simulink model "ramadan_2022"  (R2021a)
settings: Solver=ode15s  StartTime=0.0  StopTime=10  MaxStep=1e-2  MinStep=1e-20  RelTol=1e-3
StartFcn:
  | tic
StopFcn:
  | toc
  | 
  | 
  | %if GimbalLockFlag
  |  % fprintf(2, 'Almost reached Gimbal Lock of IMU. Simulation stopped.\n')
  | %end
  | 
  | %fprintf('Elapsed time: %4.2f sec (%4.2f%% realtime)\n', a, tout(end)/a*100)
values from neighbouring files (symbols this model uses):
  Balance = pMod(26:29)    [AssignSimulinkParams.m]    (also in assign_parameters.m = param(26:29))
  BalanceTrunkLat = pMod(22:25)    [AssignSimulinkParams.m]    (also in assign_parameters.m = param(22:25))
  BasisStim = pMod(1:11)    [AssignSimulinkParams.m]    (also in assign_parameters.m = param(1:11))
  CompliantLeg = pMod(12:14)    [AssignSimulinkParams.m]    (also in assign_parameters.m = param(12:14))
  CompliantLegLat = pMod(15)    [AssignSimulinkParams.m]    (also in assign_parameters.m = param(15))
  lp1 = 0.45    [nms3D_prep.m]
  lp2 = 0.55    [nms3D_prep.m]
  N = size(x,1)    [cmaes_hg.m]
  PreventKneeOverextension = pMod(16:21)    [AssignSimulinkParams.m]    (also in assign_parameters.m = param(16:21))
  propulsion = pMod(35)    [AssignSimulinkParams.m]    (also in assign_parameters.m = param(35))
  s = x(1:N-1,:).^2 + x(2:N,:).^2    [cmaes_hg.m]
  Target02 = pMod(30)    [AssignSimulinkParams.m]    (also in assign_parameters.m = param(30))
  Target13 = pMod(31:33)    [AssignSimulinkParams.m]    (also in assign_parameters.m = param(31:33))
  theta0 = pMod(34)    [AssignSimulinkParams.m]    (also in assign_parameters.m = param(34))
  WramameiSL_1000 = readmatrix('WSL_1000_Norm_Sigmoid_MSE_cont.csv')    [nms3D_prep.m]
  ZramameiSL_1000 = readmatrix('ZSL_1000_Norm_Sigmoid_MSE_cont.csv')    [nms3D_prep.m]
undefined symbols (not defined in the file or in its folder): ICs, mParams, X, Y, Z
libraries: nesl_utility x110, sm_lib x88, simulink x79, eeGeneralControl x28, robotmaniplib x10, dspinverses x10, robotcorelib x5, dspmathops x3, pid_lib x2, vrlib x1
(part 3 of 9)

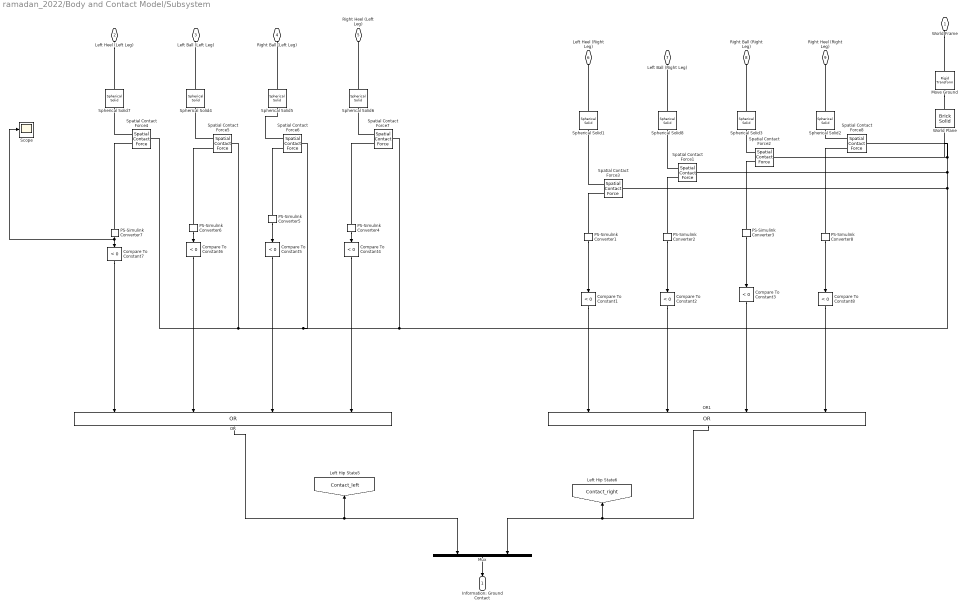
== system ramadan_2022/Body and Contact Model/Subsystem ==
  Compare To Constant{1..8} (8 alike) : simulink/Logic and Bit Operations/Compare To Constant  relop=<  const=0  OutDataTypeStr=boolean
  Move Ground : sm_lib/Frames and Transforms/Rigid Transform  TranslationMethod=StandardAxis  TranslationStandardOffset=-0.05  TranslationLengthUnit=m  TranslationStandardAxis=+Y  TranslationCartesianOffset=0  TranslationROffset=0  TranslationROffsetUnits=m  TranslationZOffset=0  TranslationZOffsetUnits=m  TranslationThetaOffset=0  TranslationThetaOffsetUnits=deg  RotationMethod=None  RotationAngleUnits=deg  RotationStandardAxis=+X  RotationAngle=-90  RotationArbitraryAxis=[0 0 1]  FollAlignAxisA=+X  BaseAlignAxisA=+Y  FollAlignAxisB=+Y  BaseAlignAxisB=+Z  RotationSequenceAxes=BaseAxes  RotationSequence=ZXZ  RotationSequenceAngles=[180 0 0]  RotationSequenceAnglesUnits=deg  RotationMatrix=[1 0 0; 0 1 0; 0 0 1]
  Mux : Mux  Inputs=2
  OR : Logic  Operator=OR  Inputs=4  AllPortsSameDT=off  OutDataTypeStr=boolean
  OR1 : Logic  Operator=OR  Inputs=4  AllPortsSameDT=off  OutDataTypeStr=boolean
  PS-Simulink Converter{1..8} (8 alike) : nesl_utility/PS-Simulink Converter  PhysicalDomain=network_engine_domain  SubClassName=ps_output  LeftPortType=input  RightPortType=output  PseudoPeriodic=off  Frequencies=[]  Unit=m  AffineConversion=off
      settings: SourceProductBaseCode=PW,SS
  Scope : Scope
  Spatial Contact Force{1..8} (8 alike) : sm_lib/Forces and Torques/Spatial Contact Force  CoefficientOfDynamicFriction=mParams.Contacts.mu_k  CoefficientOfStaticFriction=mParams.Contacts.mu_s  SenseContactBaseRotation=off  SenseContactBaseTranslation=off  NormalDamping=mParams.Contacts.damping  NormalDampingUnits=N/(m/s)  SenseContactFollowerRotation=off  SenseContactFollowerTranslation=off  SenseContactSignal=off  NormalStiffness=mParams.Contacts.stiffness  NormalStiffnessUnits=N/m  FrictionalCriticalVelocity=mParams.Contacts.vLimit  FrictionalCriticalVelocityUnits=m/s  ZeroCrossDetectContactStartAndEnd=off  FrictionType=SmoothStickSlip  SenseFrictionalForceMagnitude=off  SenseNormalForceMagnitude=off  NormalForceType=SmoothSpringDamper  SenseNormalVelocity=off  SenseSeparationDistance=on  SenseTangentialVelocity=off  SenseTangentialVelocityMagnitude=off  NormalTransitionRegionWidth=mParams.Contacts.depths  NormalTransitionRegionWidthUnits=m
  Spherical Solid{1..8} (8 alike) : sm_lib/Body Elements/Spherical Solid  GraphicAmbientColor=[0.15 0.15 0.15 1.0]  BasedOnType=Mass  CenterOfMass=[0 0 0]  CenterOfMassUnits=m  GraphicDiffuseColor=[0.5 0.5 0.5]  Density=1000  DensityUnits=kg/m^3  DoExposeReferenceFrame=on  GraphicEmissiveColor=[0.0 0.0 0.0 1.0]  ExportEntireGeometry=on  SerializedExposedGeometries=<ExposedGeometries><ExposedGeometry><RawGeometryId>entire</RawGeometryId><ExposedGeometryId>G</ExposedGeometryId></ExposedGeometry></ExposedGeometries>  SerializedFrames=<Frames/>  MarkerShape=Sphere  MarkerSize=10  GraphicType=FromGeometry  InertiaType=CalculateFromGeometry  Mass=1  MassUnits=g  MomentsOfInertia=[1 1 1]  MomentsOfInertiaUnits=kg*m^2  GraphicOpacity=1.0  ProductsOfInertia=[0 0 0]  ProductsOfInertiaUnits=kg*m^2  GraphicShininess=75  GraphicSpecularColor=[0.5 0.5 0.5 1.0]  SphereRadius=mParams.Contacts.size  SphereRadiusUnits=m  GraphicVisPropType=SimpleVisualProperties
  World Plane : sm_lib/Body Elements/Brick Solid  GraphicAmbientColor=[0.15 0.15 0.15 1.0]  BasedOnType=Density  BrickDimensions=[400 0.1 100]  BrickDimensionUnits=m  CenterOfMass=[0 0 0]  CenterOfMassUnits=m  GraphicDiffuseColor=[1.0 1.0 0.8]  Density=1000  DensityUnits=kg/(m^3)  DoExposeReferenceFrame=on  GraphicEmissiveColor=[0.0 0.0 0.0 1.0]  ExportEntireGeometry=on  SerializedFrames=<Frames/>  MarkerShape=Sphere  MarkerSize=10  GraphicType=FromGeometry  InertiaType=CalculateFromGeometry  Mass=1  MassUnits=kg  MomentsOfInertia=[1 1 1]  MomentsOfInertiaUnits=kg*m^2  GraphicOpacity=0.5  ProductsOfInertia=[0 0 0]  ProductsOfInertiaUnits=kg*m^2  GraphicShininess=75  GraphicSpecularColor=[0.5 0.5 0.5 1.0]  GraphicVisPropType=SimpleVisualProperties
  World Frame : PMIOPort  Side=Left
  Left Heel (Left Leg) : PMIOPort  Port=2  Side=Right
  Left Ball (Left Leg) : PMIOPort  Port=3  Side=Right
  Right Ball (Left Leg) : PMIOPort  Port=4  Side=Right
  Right Heel (Left Leg) : PMIOPort  Port=5  Side=Right
  Left Heel (Right Leg) : PMIOPort  Port=6  Side=Right
  Left Ball (Right Leg) : PMIOPort  Port=7  Side=Right
  Right Ball (Right Leg) : PMIOPort  Port=8  Side=Right
  Right Heel (Right Leg) : PMIOPort  Port=9  Side=Right
  Information: Ground Contact : Outport
  tag scope: Contact_left=global, Contact_right=global
  wires:
  Compare To Constant1/1 -> OR1/1
  PS-Simulink Converter4/1 -> Compare To Constant4/1
  PS-Simulink Converter5/1 -> Compare To Constant5/1
  Compare To Constant4/1 -> OR/4
  PS-Simulink Converter3/1 -> Compare To Constant3/1
  Compare To Constant6/1 -> OR/2
  PS-Simulink Converter1/1 -> Compare To Constant1/1
  PS-Simulink Converter8/1 -> Compare To Constant8/1
  Compare To Constant3/1 -> OR1/3
  Compare To Constant8/1 -> OR1/4
  PS-Simulink Converter6/1 -> Compare To Constant6/1
  PS-Simulink Converter7/1 -> Scope/1, Compare To Constant7/1
  Compare To Constant2/1 -> OR1/2
  Compare To Constant5/1 -> OR/3
  Compare To Constant7/1 -> OR/1
  PS-Simulink Converter2/1 -> Compare To Constant2/1
  OR1/1 -> [Contact_right], Mux/2
  Mux/1 -> Information: Ground Contact/1
  OR/1 -> Mux/1, [Contact_left]
  connections:
  Spatial Contact Force7/RConn1 -- Spherical Solid6/LConn1
  Spatial Contact Force5/RConn2 -- PS-Simulink Converter6/LConn1
  Spatial Contact Force1/RConn2 -- PS-Simulink Converter2/LConn1
  Spatial Contact Force7/RConn2 -- PS-Simulink Converter4/LConn1
  Spherical Solid5/RConn1 -- Right Ball (Left Leg)/RConn1
  Spatial Contact Force1/RConn1 -- Spherical Solid8/LConn1
  Spatial Contact Force2/RConn2 -- PS-Simulink Converter3/LConn1
  Spatial Contact Force8/RConn2 -- PS-Simulink Converter8/LConn1
  Spatial Contact Force6/RConn1 -- Spherical Solid5/LConn1
  Spatial Contact Force3/RConn2 -- PS-Simulink Converter1/LConn1
  Spatial Contact Force8/LConn1 -- World Plane/LConn1 -- Spatial Contact Force2/LConn1 -- Spatial Contact Force1/LConn1 -- Spatial Contact Force3/LConn1 -- Spatial Contact Force7/LConn1 -- Spatial Contact Force6/LConn1 -- Spatial Contact Force4/LConn1 -- Spatial Contact Force5/LConn1
  Spatial Contact Force5/RConn1 -- Spherical Solid4/LConn1
  Spatial Contact Force6/RConn2 -- PS-Simulink Converter5/LConn1
  Spatial Contact Force2/RConn1 -- Spherical Solid3/LConn1
  Move Ground/RConn1 -- World Plane/RConn1
  World Frame/RConn1 -- Move Ground/LConn1
  Spatial Contact Force3/RConn1 -- Spherical Solid1/LConn1
  Spherical Solid6/RConn1 -- Right Heel (Left Leg)/RConn1
  Spatial Contact Force4/RConn2 -- PS-Simulink Converter7/LConn1
  Spatial Contact Force4/RConn1 -- Spherical Solid7/LConn1
  Spherical Solid4/RConn1 -- Left Ball (Left Leg)/RConn1
  Spatial Contact Force8/RConn1 -- Spherical Solid2/LConn1
  Left Heel (Left Leg)/RConn1 -- Spherical Solid7/RConn1
  Spherical Solid2/RConn1 -- Right Heel (Right Leg)/RConn1
  Spherical Solid1/RConn1 -- Left Heel (Right Leg)/RConn1
  Spherical Solid3/RConn1 -- Right Ball (Right Leg)/RConn1
  Spherical Solid8/RConn1 -- Left Ball (Right Leg)/RConn1

== system ramadan_2022/Body and Contact Model/Trunk (floating base) ==
  Solid : sm_lib/Body Elements/Brick Solid  GraphicAmbientColor=[0.15 0.15 0.15 1.0]  BasedOnType=Density  BrickDimensions=[mParams.bodies.trunk.d mParams.bodies.trunk.l mParams.bodies.trunk.b]  BrickDimensionUnits=m  CenterOfMass=mParams.bodies.trunk.CG  CenterOfMassUnits=m  GraphicDiffuseColor=[0.5 1 0.5]  Density=2.7  DensityUnits=g/cm^3  DoExposeReferenceFrame=on  GraphicEmissiveColor=[0 0 0 1.0]  ExportEntireGeometry=off  SerializedFrames=<Frames><Frame><Id>Frame1</Id><Value><Name>CG</Name><Origin><Source>CenterOfMassFrame</Source><FeatureName></FeatureName></Origin><PrimaryAxis><DefinedDirection>+Z</DefinedDirection><Source>ReferenceFrame</Source><SourceDirection>+Z</SourceDirection><FeatureName></FeatureName></PrimaryAxis><SecondaryAxis><DefinedDirection>+X</DefinedDirection><Source>ReferenceFrame</Source><SourceDirection>+X</SourceDirection><FeatureName></FeatureName></SecondaryAxis></Value></Frame></Frames>  MarkerShape=Cube  MarkerSize=100  GraphicType=FromGeometry  InertiaType=Custom  Mass=mParams.bodies.trunk.m  MassUnits=kg  MomentsOfInertia=mParams.bodies.trunk.In  MomentsOfInertiaUnits=kg*m^2  GraphicOpacity=0.5  ProductsOfInertia=[0 0 0]  ProductsOfInertiaUnits=kg*m^2  GraphicShininess=75  GraphicSpecularColor=[0.5 0.5 0.5 1.0]  GraphicVisPropType=SimpleVisualProperties
  Transform CG to LH : sm_lib/Frames and Transforms/Rigid Transform  TranslationMethod=Cartesian  TranslationStandardOffset=0  TranslationLengthUnit=m  TranslationStandardAxis=+Y  TranslationCartesianOffset=mParams.bodies.trunk.CG_LH  TranslationROffset=0  TranslationROffsetUnits=m  TranslationZOffset=0  TranslationZOffsetUnits=m  TranslationThetaOffset=0  TranslationThetaOffsetUnits=deg  RotationMethod=None  RotationAngleUnits=deg  RotationStandardAxis=+X  RotationAngle=90  RotationArbitraryAxis=[0 0 1]  FollAlignAxisA=+X  BaseAlignAxisA=+Y  FollAlignAxisB=+Y  BaseAlignAxisB=+Z  RotationSequenceAxes=FollowerAxes  RotationSequence=XYX  RotationSequenceAngles=[0 0 0]  RotationSequenceAnglesUnits=deg  RotationMatrix=[1 0 0; 0 1 0; 0 0 1]
  Transform CG to RH : sm_lib/Frames and Transforms/Rigid Transform  TranslationMethod=Cartesian  TranslationStandardOffset=-0  TranslationLengthUnit=m  TranslationStandardAxis=+Y  TranslationCartesianOffset=mParams.bodies.trunk.CG_RH  TranslationROffset=0  TranslationROffsetUnits=m  TranslationZOffset=0  TranslationZOffsetUnits=m  TranslationThetaOffset=0  TranslationThetaOffsetUnits=deg  RotationMethod=None  RotationAngleUnits=deg  RotationStandardAxis=+X  RotationAngle=90  RotationArbitraryAxis=[0 0 1]  FollAlignAxisA=+X  BaseAlignAxisA=+Y  FollAlignAxisB=+Y  BaseAlignAxisB=+Z  RotationSequenceAxes=FollowerAxes  RotationSequence=XYX  RotationSequenceAngles=[0 0 0]  RotationSequenceAnglesUnits=deg  RotationMatrix=[1 0 0; 0 1 0; 0 0 1]
  CG : PMIOPort  Side=Left
  Left Hip : PMIOPort  Port=2  Side=Right
  Right Hip : PMIOPort  Port=3  Side=Right
  connections:
  Solid/LConn1 -- Transform CG to RH/LConn1 -- Transform CG to LH/LConn1 -- CG/RConn1
  Left Hip/RConn1 -- Transform CG to LH/RConn1
  Right Hip/RConn1 -- Transform CG to RH/RConn1

== system ramadan_2022/Body and Contact Model/Vestibular System ==
  Ankle Position Right [m] : Inport
  Ankle Position Left [m] : Inport  Port=2
  "  XYZ Sensor Left Hip" : Subsystem
  "  XYZ Sensor Right Hip" : Subsystem
  Align Axis : Subsystem
  Compare To Constant : simulink/Logic and Bit Operations/Compare To Constant  relop=<=  const=1  OutDataTypeStr=boolean
  Filtered Derivative (Discrete or Continuous) : eeGeneralControl/Filtered Derivative (Discrete or Continuous)  K=1  T=0.01  B=inf  A=-inf  minRatio=10  init_option=Inherited from block input  x0=0  Ts=0
      settings: SourceProductBaseCode=PS
  Mux : Mux  Inputs=7
  R Movement direction : Subsystem
  Scope : Scope
  Scope1 : Scope
  Selector : Selector  InputPortWidth=3  IndexOptions=Index vector (dialog)  Indices=[2]  OutputSizes=1
  Stop Simulation : Stop
  Terminator : Terminator
  Terminator1 : Terminator
  To Workspace1 : ToWorkspace  VariableName=SensorBodyFrame  SampleTime=-1
      settings: Save2DSignal=2-D array (concatenate along first dimension)
  To Workspace2 : ToWorkspace  VariableName=xyzHAT  SampleTime=-1
      settings: Save2DSignal=2-D array (concatenate along first dimension)
  "Trunk Sensor " : Subsystem
  frame : PMIOPort  Side=Left
  Right Hip : PMIOPort  Port=2  Side=Left
  Left Hip : PMIOPort  Port=3  Side=Left
  tag scope: AnklePosL_rot=global, AnklePosR_rot=global, CoM_Position=global, CoM_Velocity=global, CoM_Velocity_rot=global, HeelPosL_rot=global, HeelPosR_rot=global, HipL=global, HipR=global, R_body=global, RotationTrunk=global, RotationVelocityTrunk=global, TRK_CG=global, TrunkRotVel_lat=global, TrunkRotVel_sag=global, TrunkRot_lat=global, TrunkRot_sag=global
  wires:
  Selector/1 -> Compare To Constant/1
  Compare To Constant/1 -> Stop Simulation/1
  "Trunk Sensor "/2(Velocity Trunk [m/s]) -> Align Axis/5(Velocity Trunk [m/s]), Scope/1, Filtered Derivative (Discrete or Continuous)/1, [CoM_Velocity]
  "Trunk Sensor "/4(Rotation Trunk [rad]) -> [RotationTrunk]
  Ankle Position Right [m]/1 -> Align Axis/1(Ankle Position Right [m])
  "  XYZ Sensor Right Hip"/1(Hip Position [m]) -> [HipR], R Movement direction/1(Hip Right), Align Axis/7(Hip Position Right [m])
  R Movement direction/1("R ") -> [R_body], Align Axis/3("R ")
  Ankle Position Left [m]/1 -> Align Axis/2(Ankle Position Left [m])
  "Trunk Sensor "/1(Position Trunk [m]) -> [TRK_CG], Selector/1, To Workspace2/1, Align Axis/4(Position Trunk [m]), [CoM_Position]
  "  XYZ Sensor Left Hip"/1(Hip Position [m]) -> [HipL], Align Axis/6(Hip Position Left [m]), R Movement direction/2(Hip Left)
  "Trunk Sensor "/3(Rotation Velocity Trunk [rad/s]) -> [RotationVelocityTrunk]
  Mux/1 -> To Workspace1/1
  "  XYZ Sensor Right Hip"/2(Hip Velocity [m/s]) -> Terminator/1
  "  XYZ Sensor Left Hip"/2(Hip Velocity [m/s]) -> Terminator1/1
  Align Axis/1(Ankle Position Left (body frame)) -> [AnklePosL_rot], Mux/1
  Align Axis/2(Ankle Position Right (body frame)) -> Scope1/1, [AnklePosR_rot], Mux/2
  Align Axis/3(Trunk Velocity (body frame)) -> [CoM_Velocity_rot], Mux/3
  Align Axis/4(Saggital Trunk Rotation [rad] (body frame)) -> [TrunkRot_sag], Mux/4
  Align Axis/5(Lateral Trunk Rotation [rad] (body frame)) -> [TrunkRot_lat], Mux/5
  Align Axis/6(Saggital Trunk Rotation Velocity [rad/s] (body frame)) -> [TrunkRotVel_sag], Mux/6
  Align Axis/7(Lateral Trunk Rotation Velocity [rad/s] (body frame)) -> [TrunkRotVel_lat], Mux/7
  Align Axis/8(Heel Position Left (body frame)) -> [HeelPosL_rot]
  Align Axis/9(Heel Position Right (body frame)) -> [HeelPosR_rot]
  connections:
  "Trunk Sensor "/LConn1 -- frame/RConn1
  "  XYZ Sensor Left Hip"/LConn1 -- Left Hip/RConn1
  "  XYZ Sensor Right Hip"/LConn1 -- Right Hip/RConn1

== system ramadan_2022/Body and Contact Model/World Frame ==
  Mechanism Configuration : sm_lib/Utilities/Mechanism Configuration  UniformGravity=Constant  GravityVector=[0 -9.81 0]  GravityVectorUnits=m/s^2  GravityUnits=m/s^2  LinearizationDelta=0.001  JointModeTransitionNonlinearIterations=2
  Solver Configuration : nesl_utility/Solver Configuration  PhysicalDomain=network_engine_domain  SubClassName=solver  LeftPortType=input  RightPortType=generic  Tones=[]  Harmonics=[]  SimulateNoise=off  Profile=off  UseLocalSampling=off  EnableSwitchedLinearOptims=on  FrequencyDomain=off  UseCCode=off  RelTol=0.001  AbsTol=1e-06  MinStep=1e-09  ToWorkspace=off  RevertToSquareIcSolve=off  NumHomotopyIterations=100  PhasorMode=off  PhasorModeNumHarmonics=1  DoDC=off  ResidualTolerance=1e-9  UseLocalSolver=off  LocalSolverChoice=NE_BACKWARD_EULER_ADVANCER  LocalSolverSampleTime=.001  DoFixedCost=off  MaxNonlinIter=3  MaxModeIter=2  ComputeImpulses=off  ImpulseIterations=2  LinearAlgebra=Sparse  EquationFormulation=NE_TIME_EF  DelaysMemoryBudget=1024  AutomaticFiltering=on  FilteringTimeConstant=0.001  PartitionStorageMethod=AS_NEEDED  PartitionMemoryBudget=1024  PartitionMethod=FAST
      settings: SourceProductBaseCode=PW,SS
  World Frame : sm_lib/Frames and Transforms/World Frame
  Conn1 : PMIOPort  Side=Right
  connections:
  Solver Configuration/RConn1 -- Mechanism Configuration/RConn1 -- Conn1/RConn1 -- World Frame/RConn1

== system ramadan_2022/CMA Data/SS_dist1 ==
  In1 : Inport
  Trigger : TriggerPort  VariantControl=(inherit)  ZeroCross=off
  Delay : Delay
  Delay1 : Delay  DelayLength=1
  Mux : Mux  Inputs=3
  To Current Workspace4 : ToWorkspace  VariableName=SSdist  SaveFormat=Structure With Time  SampleTime=-1
      settings: MaxDataPoints=3
  SSdist : Outport
  wires:
  In1/1 -> Delay/1, Delay1/1, Mux/3, To Current Workspace4/1
  Delay/1 -> Mux/1
  Delay1/1 -> Mux/2
  Mux/1 -> SSdist/1

== system ramadan_2022/CMA Data/SS_dist2 ==
  Steplengths : Inport
  Trigger : TriggerPort  VariantControl=(inherit)  ZeroCross=off
  Steplength at DS : Outport
  wires:
  Steplengths/1 -> Steplength at DS/1

== system ramadan_2022/CMA Data/Step Counter ==
  Step2 : Inport
  Step1 : Inport  Port=2
  Constant1 : Constant  Value=0
  Constant2 : Constant  Value=0
  Constant3 : Constant  Value=0
  Constant4 : Constant  Value=-1
  Saturation Dynamic : simulink/Discontinuities/Saturation Dynamic  OutMin=[]  OutMax=[]  OutDataTypeStr=Inherit: Same as second input  OutDataType=fixdt(1, 16)  OutScaling=2^-10  DoSatur=off
  Saturation Dynamic1 : simulink/Discontinuities/Saturation Dynamic  OutMin=[]  OutMax=[]  OutDataTypeStr=Inherit: Same as second input  OutDataType=fixdt(1, 16)  OutScaling=2^-10  DoSatur=off
  Sum : Sum  Inputs=|++
  Sum1 : Sum  Inputs=++|
  Sum2 : Sum  Inputs=|++
  count steps1 : Subsystem  TreatAsAtomicUnit=on
  count steps2 : Subsystem  TreatAsAtomicUnit=on
  nStep : Outport  VectorParamsAs1DForOutWhenUnconnected=off
  wires:
  count steps1/1(nStep) -> Saturation Dynamic1/2, Sum2/2, Sum/2
  count steps2/1(nStep) -> Saturation Dynamic/2, Sum1/1, Sum/1
  Constant3/1 -> Saturation Dynamic/3
  Saturation Dynamic/1 -> count steps2/1(nStep-1)
  Constant1/1 -> Sum1/2
  Sum1/1 -> Saturation Dynamic1/1
  Constant2/1 -> Saturation Dynamic1/3
  Saturation Dynamic1/1 -> count steps1/1(nStep-1)
  Constant4/1 -> Sum2/1
  Sum2/1 -> Saturation Dynamic/1
  Step2/1 -> count steps2/Trigger
  Sum/1 -> nStep/1
  Step1/1 -> count steps1/Trigger

== system ramadan_2022/CMA Data/Triggered Subsystem ==
  In1 : Inport
  Trigger : TriggerPort  VariantControl=Variant
  Out1 : Outport
  wires:
  In1/1 -> Out1/1

== system ramadan_2022/CMA Data/check steady state ==
  p : Inport
  nStep : Inport  Port=2
  Abs : Abs  ZeroCross=off
  Add{,1..9,15..16} (12 alike) : Sum  Inputs=-+
  Add{10..14,17} (6 alike) : Sum  Inputs=+-
  Demux2 : Demux  Outputs=7
  Demux3 : Demux  Outputs=7
  Fcn : Fcn  Expr=rem(u(1), 2)
  Gain14 : Gain  Gain=.5
  Mux1 : Mux  Inputs=6
  Rounding Function1 : Rounding
  Sum of Elements : Sum  Inputs=+
  even : Subsystem  TreatAsAtomicUnit=on
  odd : Subsystem  TreatAsAtomicUnit=on
  SS_dist : Outport  VectorParamsAs1DForOutWhenUnconnected=off
  wires:
  p/1 -> even/1(In1), odd/1(In1)
  Fcn/1 -> odd/Trigger, even/Trigger
  odd/1(Out1) -> Demux2/1
  even/1(Out1) -> Demux3/1
  Add10/1 -> Mux1/1
  Add11/1 -> Mux1/2
  Add12/1 -> Mux1/3
  Add13/1 -> Mux1/4
  Add14/1 -> Mux1/5
  Demux2/2 -> Add/2
  Demux2/3 -> Add1/2
  Demux2/4 -> Add2/2
  Demux2/5 -> Add3/2
  Demux2/6 -> Add4/2
  Demux2/1 -> Add/1, Add1/1, Add2/1, Add3/1, Add4/1, Add15/1
  Demux3/2 -> Add5/2
  Demux3/3 -> Add6/2
  Demux3/4 -> Add7/2
  Demux3/5 -> Add8/2
  Demux3/6 -> Add9/2
  Demux3/1 -> Add5/1, Add6/1, Add7/1, Add8/1, Add9/1, Add16/1
  Add/1 -> Add10/1
  Add1/1 -> Add11/1
  Add2/1 -> Add12/1
  Add3/1 -> Add13/1
  Add4/1 -> Add14/1
  Add5/1 -> Add10/2
  Add6/1 -> Add11/2
  Add7/1 -> Add12/2
  Add8/1 -> Add13/2
  Add9/1 -> Add14/2
  Mux1/1 -> Abs/1
  Abs/1 -> Sum of Elements/1
  Sum of Elements/1 -> SS_dist/1
  nStep/1 -> Gain14/1
  Gain14/1 -> Rounding Function1/1
  Rounding Function1/1 -> Fcn/1
  Demux2/7 -> Add15/2
  Demux3/7 -> Add16/2
  Add15/1 -> Add17/1
  Add16/1 -> Add17/2
  Add17/1 -> Mux1/6

== system ramadan_2022/CMA Data/mean (10s) ==
  u : Inport
  Constant : Constant  Value=1001
  Divide2 : Product  Inputs=*/
  Sum of Elements : Sum  Inputs=+  CollapseMode=Specified dimension  AccumDataTypeStr=double
  Tapped Delay : simulink/Discrete/Tapped Delay  vinit=1  samptime=0.01  NumDelays=1000  DelayOrder=Newest  includeCurrent=off
  Vector Concatenate : Concatenate
  u_average : Outport
  wires:
  Tapped Delay/1 -> Vector Concatenate/2
  Vector Concatenate/1 -> Sum of Elements/1
  Sum of Elements/1 -> Divide2/1
  Divide2/1 -> u_average/1
  u/1 -> Tapped Delay/1, Vector Concatenate/1
  Constant/1 -> Divide2/2

== system ramadan_2022/CMA Data/mean (10s)1 ==
  u : Inport
  Constant : Constant  Value=1001
  Divide2 : Product  Inputs=*/
  Sum of Elements : Sum  Inputs=+  CollapseMode=Specified dimension  AccumDataTypeStr=double
  Tapped Delay : simulink/Discrete/Tapped Delay  vinit=ICs.trunk.vx0  samptime=0.01  NumDelays=1000  DelayOrder=Newest  includeCurrent=off
  Vector Concatenate : Concatenate
  u_average : Outport
  wires:
  Tapped Delay/1 -> Vector Concatenate/2
  Vector Concatenate/1 -> Sum of Elements/1
  Sum of Elements/1 -> Divide2/1
  Divide2/1 -> u_average/1
  u/1 -> Tapped Delay/1, Vector Concatenate/1
  Constant/1 -> Divide2/2

== system ramadan_2022/CMA Data/mean (10s)2 ==
  u : Inport
  Constant : Constant  Value=1001
  Divide2 : Product  Inputs=*/
  Sum of Elements : Sum  Inputs=+  CollapseMode=Specified dimension  AccumDataTypeStr=double
  Tapped Delay : simulink/Discrete/Tapped Delay  vinit=ICs.trunk.vx0  samptime=0.001  NumDelays=1000  DelayOrder=Newest  includeCurrent=off
  Vector Concatenate : Concatenate
  u_average : Outport
  wires:
  Tapped Delay/1 -> Vector Concatenate/2
  Vector Concatenate/1 -> Sum of Elements/1
  Sum of Elements/1 -> Divide2/1
  Divide2/1 -> u_average/1
  u/1 -> Tapped Delay/1, Vector Concatenate/1
  Constant/1 -> Divide2/2

== system ramadan_2022/CMA Data/phase 1? ==
  cadence : Inport
  stability : Inport  Port=2
  AND1 : Logic  AllPortsSameDT=off  OutDataTypeStr=boolean
  AND2 : Logic  AllPortsSameDT=off  OutDataTypeStr=boolean
  Clock : Clock
  Compare To Constant : simulink/Logic and Bit Operations/Compare To Constant  relop=>=  const=30  OutDataTypeStr=boolean
  Compare To Constant1 : simulink/Logic and Bit Operations/Compare To Constant  relop=<=  const=135  OutDataTypeStr=boolean
  Compare To Constant2 : simulink/Logic and Bit Operations/Compare To Constant  relop===  const=10  OutDataTypeStr=boolean
  OR : Logic  Operator=OR  AllPortsSameDT=off  OutDataTypeStr=boolean
  Stop Simulation1 : Stop
  time : Outport
  wires:
  cadence/1 -> Compare To Constant1/1
  Compare To Constant1/1 -> AND1/1
  Compare To Constant/1 -> AND2/2
  stability/1 -> Compare To Constant/1
  Compare To Constant2/1 -> AND2/1, AND1/2
  AND2/1 -> OR/2
  AND1/1 -> OR/1
  Clock/1 -> time/1, Compare To Constant2/1
  OR/1 -> Stop Simulation1/1

== system ramadan_2022/Muscle Actuation Layer/Muscles Left ==
  STIM Left : Inport
  Demux : Demux
  Muscle Dynamics (Vectorized)1 : Subsystem
  Muscle Length Vector1 : Subsystem
  Muscle Torque Contributions1 : Subsystem
  Terminator : Terminator
  Terminator1 : Terminator
  To Workspace1 : ToWorkspace  VariableName=LForce  SampleTime=-1
      settings: Save2DSignal=2-D array (concatenate along first dimension)
  tauHipPitchL : Outport
  tauHipRollL : Outport  Port=2
  tauKneeL : Outport  Port=3
  tauHipAnkleL : Outport  Port=4
  "Leg Torque " : Outport  Port=5
  tag scope: LFmVec=global, LLceVec=global, LVceVec=global
  wires:
  Demux/2 -> Muscle Length Vector1/2(qHipRoll [rad])
  Muscle Torque Contributions1/2(tauHR [Nm]) -> tauHipRollL/1
  Demux/1 -> Muscle Length Vector1/1(qHipPitch [rad])
  Demux/4 -> Muscle Torque Contributions1/2(qAnkle [rad]), Muscle Length Vector1/4(qAnkle [rad])  "qA"
  Muscle Dynamics (Vectorized)1/3(Vce) -> [LVceVec]
  Muscle Torque Contributions1/3(tauK [Nm]) -> tauKneeL/1
  Demux/3 -> Muscle Torque Contributions1/1(qKnee [rad]), Muscle Length Vector1/3(qKnee [rad])  "qK"
  Muscle Dynamics (Vectorized)1/5(ForceLengthFactor) -> Terminator1/1
  Muscle Length Vector1/1(lmtc [m x11]) -> Muscle Dynamics (Vectorized)1/1(lmtc [m])
  Muscle Torque Contributions1/1(tauHP [Nm]) -> tauHipPitchL/1
  Muscle Torque Contributions1/4(tauA [Nm]) -> tauHipAnkleL/1
  Muscle Dynamics (Vectorized)1/4(A) -> Terminator/1
  Muscle Dynamics (Vectorized)1/2(Lce) -> [LLceVec]
  STIM Left/1 -> Muscle Dynamics (Vectorized)1/2(STIM)
  [Llegq] -> Demux/1
  Muscle Torque Contributions1/5(Leg Torque) -> "Leg Torque "/1
  Muscle Dynamics (Vectorized)1/1(Fmtc) -> To Workspace1/1, Muscle Torque Contributions1/3(FmVec [N x11]), [LFmVec]

== system ramadan_2022/Muscle Actuation Layer/Muscles Right ==
  STIM Right : Inport
  Demux : Demux
  Goto15 : Goto  Commented=on  GotoTag=activation_R  TagVisibility=global
  Muscle Dynamics (Vectorized) : Subsystem
  Muscle Length Vector : Subsystem
  Muscle Torque Contributions : Subsystem
  R Leg Muscles Vce [m/s x11]1 : Goto  Commented=on  GotoTag=RForceLength  TagVisibility=global
  To Workspace1 : ToWorkspace  VariableName=RForce  SampleTime=-1
      settings: Save2DSignal=2-D array (concatenate along first dimension)
  tauHipPitchR : Outport
  tauHipRollR : Outport  Port=2
  tauKneeR : Outport  Port=3
  tauHipAnkleR : Outport  Port=4
  Leg Torque : Outport  Port=5
  tag scope: RFmVec=global, RLceVec=global, RVceVec=global
  wires:
  Muscle Torque Contributions/4(tauA [Nm]) -> tauHipAnkleR/1
  Muscle Torque Contributions/3(tauK [Nm]) -> tauKneeR/1
  Muscle Length Vector/1(lmtc [m x11]) -> Muscle Dynamics (Vectorized)/1(lmtc [m])
  Demux/3 -> Muscle Torque Contributions/1(qKnee [rad]), Muscle Length Vector/3(qKnee [rad])  "qK"
  Demux/4 -> Muscle Torque Contributions/2(qAnkle [rad]), Muscle Length Vector/4(qAnkle [rad])  "qA"
  Muscle Dynamics (Vectorized)/2(Lce) -> [RLceVec]
  Muscle Torque Contributions/2(tauHR [Nm]) -> tauHipRollR/1
  Demux/1 -> Muscle Length Vector/1(qHipPitch [rad])  "qHP"
  Muscle Dynamics (Vectorized)/5(ForceLengthFactor) -> R Leg Muscles Vce [m/s x11]1/1
  Muscle Dynamics (Vectorized)/1(Fmtc) -> To Workspace1/1, Muscle Torque Contributions/3(FmVec [N x11]), [RFmVec]
  Muscle Dynamics (Vectorized)/4(A) -> Goto15/1
  Muscle Dynamics (Vectorized)/3(Vce) -> [RVceVec]
  Muscle Torque Contributions/1(tauHP [Nm]) -> tauHipPitchR/1
  Demux/2 -> Muscle Length Vector/2(qHipRoll [rad])  "qHR"
  STIM Right/1 -> Muscle Dynamics (Vectorized)/2(STIM)
  [Rlegq] -> Demux/1  "qHP"
  Muscle Torque Contributions/5(Leg Torque) -> Leg Torque/1

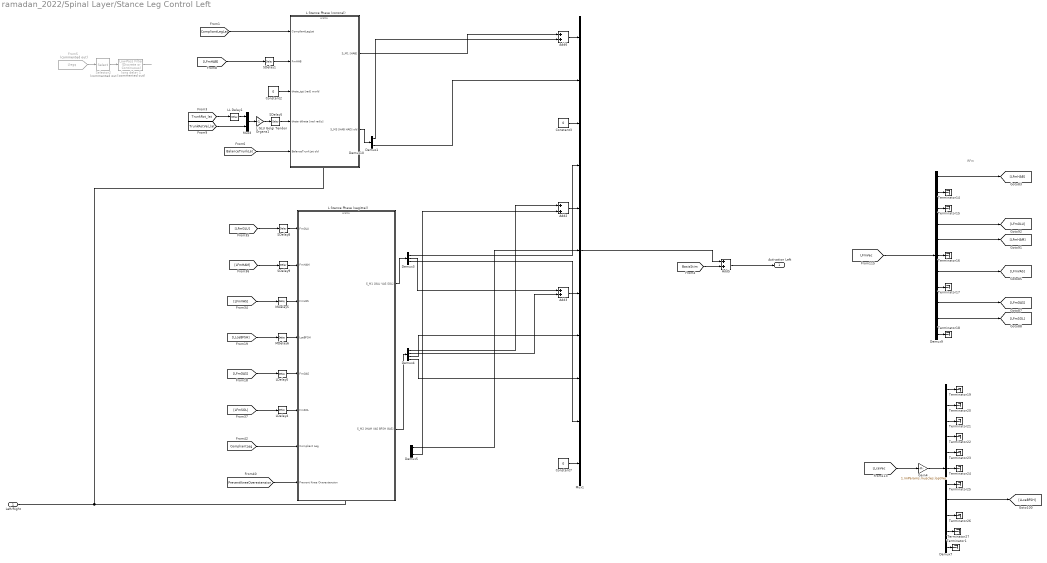
== system ramadan_2022/Spinal Layer/Stance Leg Control Left ==
  note: RFm
  Left/Right : Inport
  Add{2..3,5..6} (4 alike) : Sum
  Constant2 : Constant  Value=0
  Constant3 : Constant  Value=0
  Constant7 : Constant  Value=0
  Demux1 : Demux  Outputs=2
  Demux10 : Demux  Outputs=2
  Demux3 : Demux  Outputs=3
  Demux4 : Demux
  Demux5 : Demux  Outputs=2
  Demux7 : Demux  Outputs=11
  Demux9 : Demux  Outputs=11
  From5 : From  Commented=on  GotoTag=Llegq  TagVisibility=global
      settings: CloseFcn=tagdialog Close
  Gain4 : Gain  Gain=1./mParams.muscles.loptVec
  L GLU Golgi Tendon Organs1 : Gain  Gain=-1
  L Stance Phase (coronal) : Subsystem  TreatAsAtomicUnit=on
  L Stance Phase (sagittal) : Subsystem  TreatAsAtomicUnit=on
  LDelay4 : TransportDelay  DelayTime=mParams.control.delays.long
  LDelay5 : TransportDelay  DelayTime=mParams.control.delays.long
  LL Delay1 : TransportDelay  DelayTime=mParams.control.delays.longloop/2
  MDelay5 : TransportDelay  DelayTime=mParams.control.delays.mid
  MDelay6 : TransportDelay  DelayTime=mParams.control.delays.mid
  Mux1 : Mux  Inputs=11
  Mux3 : Mux  Inputs=2
  SDelay{1,5,8..9} (4 alike) : TransportDelay  DelayTime=mParams.control.delays.short
  Selector2 : Selector  Commented=on  InputPortWidth=4  IndexOptions=Index vector (dialog)  Indices=[2]  OutputSizes=1
  Terminator{1,14..27} (15 alike) : Terminator
  long delay 1 : eeGeneralControl/Low-Pass Filter (Discrete or Continuous)  Commented=on  K=1  T=0.005  B=inf  A=-inf  init_option=Inherited from block input  x0=0  Ts=0
  Activation Left : Outport
  wires:
  [LFmVec] -> Demux9/1
  Demux9/1 -> [LFmHAB]
  Gain4/1 -> Demux7/1
  Demux9/5 -> [LFmHAM]
  Demux7/8 -> [LLceBFSH]
  [LLceVec] -> Gain4/1
  Demux9/9 -> [LFmGAS]
  Demux9/10 -> [LFmSOL]
  Demux9/4 -> [LFmGLU]
  Demux9/7 -> [LFmVAS]
  Demux7/11 -> Terminator1/1
  Add5/1 -> Activation Left/1
  Left/Right/1 -> L Stance Phase (sagittal)/Enable, L Stance Phase (coronal)/Enable
  Demux9/2 -> Terminator14/1
  Demux9/3 -> Terminator15/1
  Demux9/6 -> Terminator16/1
  Demux9/8 -> Terminator17/1
  Demux9/11 -> Terminator18/1
  Demux7/1 -> Terminator19/1
  Demux7/2 -> Terminator20/1
  Demux7/3 -> Terminator21/1
  Demux7/4 -> Terminator22/1
  Demux7/5 -> Terminator23/1
  Demux7/6 -> Terminator24/1
  Demux7/7 -> Terminator25/1
  Demux7/9 -> Terminator26/1
  Demux7/10 -> Terminator27/1
  [BasisStim] -> Add5/2
  Mux1/1 -> Add5/1
  Constant7/1 -> Mux1/11
  Add2/1 -> Mux1/5
  Add3/1 -> Mux1/7
  [LFmGLU] -> SDelay8/1
  SDelay9/1 -> L Stance Phase (sagittal)/2(FmHAM)
  MDelay6/1 -> L Stance Phase (sagittal)/4(LceBFSH)
  [LLceBFSH] -> MDelay6/1
  [LFmSOL] -> LDelay4/1
  MDelay5/1 -> L Stance Phase (sagittal)/3(FmVAS)
  [LFmGAS] -> LDelay5/1
  LDelay5/1 -> L Stance Phase (sagittal)/5(FmGAS)
  SDelay8/1 -> L Stance Phase (sagittal)/1(FmGLU)
  [LFmHAM] -> SDelay9/1
  LDelay4/1 -> L Stance Phase (sagittal)/6(FmSOL)
  [LFmVAS] -> MDelay5/1
  [CompliantLeg] -> L Stance Phase (sagittal)/7(Compliant Leg)
  [PreventKneeOverextension] -> L Stance Phase (sagittal)/8(Prevent Knee Overextension)
  [CompliantLegLat] -> L Stance Phase (coronal)/1(CompliantLegLat)
  From5/1 -> Selector2/1
  [LFmHAB] -> SDelay1/1
  SDelay1/1 -> L Stance Phase (coronal)/2(FmHAB)
  long delay 1/1 -> ?
  Add6/1 -> Mux1/1
  Selector2/1 -> long delay 1/1
  SDelay5/1 -> L Stance Phase (coronal)/4(theta dtheta [rad rad/s])
  [TrunkRotVel_lat] -> Mux3/2
  [TrunkRot_lat] -> LL Delay1/1
  LL Delay1/1 -> Mux3/1
  [BalanceTrunkLat] -> L Stance Phase (coronal)/5(BalanceTrunkLat old)
  Mux3/1 -> L GLU Golgi Tendon Organs1/1
  L GLU Golgi Tendon Organs1/1 -> SDelay5/1
  L Stance Phase (coronal)/1(S_M1 [HAB]) -> Add6/1
  L Stance Phase (coronal)/2(S_M3 [HAB HAD] old) -> Demux1/1
  Demux1/1 -> Add6/2
  Demux1/2 -> Mux1/2
  L Stance Phase (sagittal)/1(S_M1 [GLU VAS SOL]) -> Demux3/1
  L Stance Phase (sagittal)/2(S_M2 [HAM VAS BFSH GAS]) -> Demux4/1
  ? -> Demux5/1
  Demux3/1 -> Mux1/4
  Demux4/1 -> Add2/1
  Demux5/2 -> Add2/2
  Demux5/1 -> Mux1/6
  Demux3/2 -> Add3/1
  Demux4/2 -> Add3/2
  Demux4/3 -> Mux1/8
  Demux4/4 -> Mux1/9
  Demux3/3 -> Mux1/10
  Constant2/1 -> L Stance Phase (coronal)/3(theta_tgt [rad] world)
  Constant3/1 -> Mux1/3

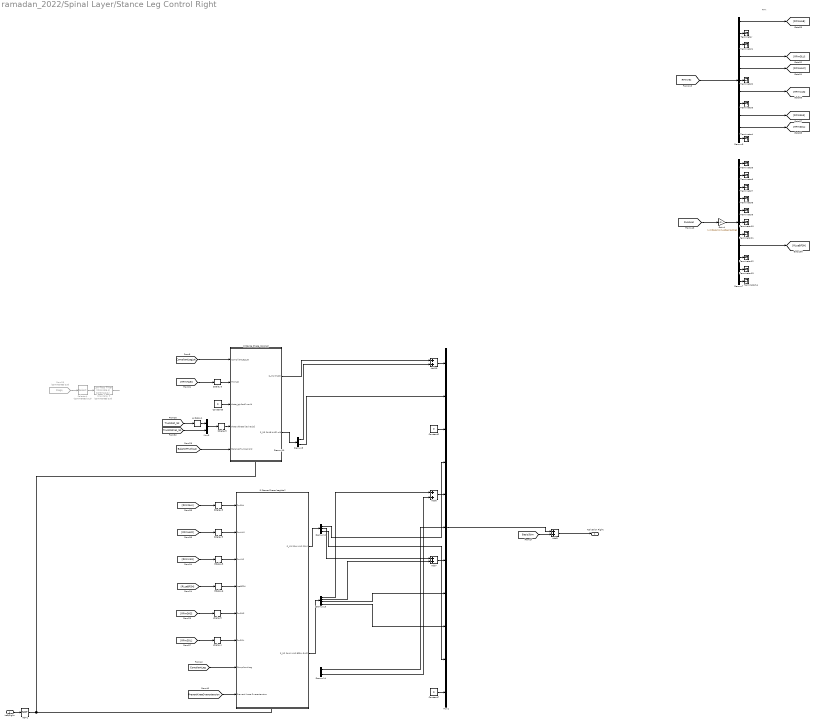
== system ramadan_2022/Spinal Layer/Stance Leg Control Right ==
  note: RFm
  Left/Right : Inport
  Add{6..7,9..10} (4 alike) : Sum
  Constant2 : Constant  Value=0
  Constant3 : Constant  Value=0
  Constant7 : Constant  Value=0
  Demux10 : Demux  Outputs=2
  Demux12 : Demux  Outputs=3
  Demux13 : Demux
  Demux14 : Demux  Outputs=2
  Demux7 : Demux  Outputs=11
  Demux8 : Demux  Outputs=2
  Demux9 : Demux  Outputs=11
  From28 : From  Commented=on  GotoTag=Rlegq  TagVisibility=global
      settings: CloseFcn=tagdialog Close
  Gain4 : Gain  Gain=1./mParams.muscles.loptVec
  LDelay4 : TransportDelay  DelayTime=mParams.control.delays.long
  LDelay5 : TransportDelay  DelayTime=mParams.control.delays.long
  LL Delay1 : TransportDelay  DelayTime=mParams.control.delays.longloop/2
  MDelay5 : TransportDelay  DelayTime=mParams.control.delays.mid
  MDelay6 : TransportDelay  DelayTime=mParams.control.delays.mid
  Mux1 : Mux  Inputs=11
  Mux3 : Mux  Inputs=2
  NOT1 : Logic  Operator=NOT  AllPortsSameDT=off  OutDataTypeStr=boolean
  R Stance Phase (coronal) : Subsystem  TreatAsAtomicUnit=on
  R Stance Phase (sagittal) : Subsystem  TreatAsAtomicUnit=on
  SDelay{3,5,8..9} (4 alike) : TransportDelay  DelayTime=mParams.control.delays.short
  Selector4 : Selector  Commented=on  InputPortWidth=4  IndexOptions=Index vector (dialog)  Indices=[2]  OutputSizes=1
  Terminator{,1..14} (15 alike) : Terminator
  long delay 3 : eeGeneralControl/Low-Pass Filter (Discrete or Continuous)  Commented=on  K=1  T=0.005  B=inf  A=-inf  init_option=Inherited from block input  x0=0  Ts=0
  Activation Right : Outport
  wires:
  [RFmVec] -> Demux9/1
  Demux9/1 -> [RFmHAB]
  Gain4/1 -> Demux7/1
  Demux9/5 -> [RFmHAM]
  Demux7/8 -> [RLceBFSH]
  Demux9/9 -> [RFmGAS]
  Demux9/10 -> [RFmSOL]
  Demux9/4 -> [RFmGLU]
  Demux9/7 -> [RFmVAS]
  Demux7/11 -> Terminator14/1
  [RLceVec] -> Gain4/1
  Demux9/2 -> Terminator/1
  Demux9/3 -> Terminator1/1
  Demux9/6 -> Terminator2/1
  Demux9/8 -> Terminator3/1
  Demux9/11 -> Terminator4/1
  Demux7/1 -> Terminator5/1
  Demux7/2 -> Terminator6/1
  Demux7/3 -> Terminator7/1
  Demux7/4 -> Terminator8/1
  Demux7/5 -> Terminator9/1
  Demux7/6 -> Terminator10/1
  Demux7/7 -> Terminator11/1
  Demux7/9 -> Terminator12/1
  Demux7/10 -> Terminator13/1
  [RFmHAB] -> SDelay3/1
  LL Delay1/1 -> Mux3/1
  [CompliantLeg] -> R Stance Phase (sagittal)/7(Compliant Leg)
  Demux13/1 -> Add6/1
  Left/Right/1 -> NOT1/1
  Demux12/2 -> Add7/1
  [RFmGLU] -> SDelay8/1
  SDelay8/1 -> R Stance Phase (sagittal)/1(FmGLU)
  [RLceBFSH] -> MDelay6/1
  Add6/1 -> Mux1/5
  Demux12/3 -> Mux1/10
  MDelay6/1 -> R Stance Phase (sagittal)/4(LceBFSH)
  Mux3/1 -> SDelay5/1
  From28/1 -> Selector4/1
  Demux13/4 -> Mux1/9
  [RFmGAS] -> LDelay5/1
  Constant7/1 -> Mux1/11
  [RFmSOL] -> LDelay4/1
  SDelay9/1 -> R Stance Phase (sagittal)/2(FmHAM)
  [TrunkRot_lat] -> LL Delay1/1
  LDelay4/1 -> R Stance Phase (sagittal)/6(FmSOL)
  [BasisStim] -> Add9/2
  Add10/1 -> Mux1/1
  Add7/1 -> Mux1/7
  Mux1/1 -> Add9/1
  Constant2/1 -> Mux1/3
  Add9/1 -> Activation Right/1
  R Stance Phase (coronal)/1(S_M1 [HAB]) -> Add10/1
  ? -> Demux14/1
  [RFmVAS] -> MDelay5/1
  Demux13/2 -> Add7/2
  Demux13/3 -> Mux1/8
  Selector4/1 -> long delay 3/1
  Demux14/2 -> Add6/2
  R Stance Phase (coronal)/2(S_M3 [HAB HAD] old) -> Demux8/1
  Demux14/1 -> Mux1/6
  Demux8/2 -> Mux1/2
  [RFmHAM] -> SDelay9/1
  Demux12/1 -> Mux1/4
  long delay 3/1 -> ?
  SDelay5/1 -> R Stance Phase (coronal)/4(theta dtheta [rad rad/s])
  R Stance Phase (sagittal)/2(S_M2 [HAM VAS BFSH GAS]) -> Demux13/1
  R Stance Phase (sagittal)/1(S_M1 [GLU VAS SOL]) -> Demux12/1
  Demux8/1 -> Add10/2
  LDelay5/1 -> R Stance Phase (sagittal)/5(FmGAS)
  [PreventKneeOverextension] -> R Stance Phase (sagittal)/8(Prevent Knee Overextension)
  MDelay5/1 -> R Stance Phase (sagittal)/3(FmVAS)
  [TrunkRotVel_lat] -> Mux3/2
  [BalanceTrunkLat] -> R Stance Phase (coronal)/5(BalanceTrunkLat old)
  [CompliantLegLat] -> R Stance Phase (coronal)/1(CompliantLegLat)
  SDelay3/1 -> R Stance Phase (coronal)/2(FmHAB)
  NOT1/1 -> R Stance Phase (sagittal)/Enable, R Stance Phase (coronal)/Enable
  Constant3/1 -> R Stance Phase (coronal)/3(theta_tgt [rad] world)

== system ramadan_2022/Spinal Layer/Stretch Reflex for Swing Leg Control ==
  Descending Commands Left : Inport
  Descending Commands Right : Inport  Port=2
  Filtered Derivative (Discrete or Continuous)1 : eeGeneralControl/Filtered Derivative (Discrete or Continuous)  K=1  T=0.0025  B=inf  A=-inf  minRatio=10  init_option=Inherited from block input  x0=0  Ts=0
      settings: SourceProductBaseCode=PS
  Filtered Derivative (Discrete or Continuous)2 : eeGeneralControl/Filtered Derivative (Discrete or Continuous)  K=1  T=0.0025  B=inf  A=-inf  minRatio=10  init_option=Inherited from block input  x0=0  Ts=0
      settings: SourceProductBaseCode=PS
  Saturation1 : Saturate  UpperLimit=1  LowerLimit=0  ZeroCross=off
  Saturation4 : Saturate  UpperLimit=1  LowerLimit=0  ZeroCross=off
  Stretch Reflex Left : Subsystem
  Stretch Reflex Right : Subsystem
  Time Delay{,1..4} (5 alike) : eeGeneralControl/Low-Pass Filter (Discrete or Continuous)  K=1  T=0.0025  B=inf  A=-inf  init_option=Inherited from block input  x0=0  Ts=0
  Time Delay5 : eeGeneralControl/Low-Pass Filter (Discrete or Continuous)  K=1  T=0.0025  B=inf  A=-inf  init_option=Inherited from block input  x0=0  Ts=-1
  Activation Left : Outport
  Activation Right : Outport  Port=2
  wires:
  Descending Commands Left/1 -> Time Delay/1, Filtered Derivative (Discrete or Continuous)2/1
  Filtered Derivative (Discrete or Continuous)1/1 -> Stretch Reflex Right/4(lambda_dot)
  Descending Commands Right/1 -> Time Delay3/1, Filtered Derivative (Discrete or Continuous)1/1
  Stretch Reflex Right/1(STIM) -> Saturation4/1
  Stretch Reflex Left/1(STIM) -> Saturation1/1
  Filtered Derivative (Discrete or Continuous)2/1 -> Stretch Reflex Left/4(lambda_dot)
  [LLceVec] -> Time Delay1/1
  [LVceVec] -> Time Delay2/1
  [RVceVec] -> Time Delay5/1
  [RLceVec] -> Time Delay4/1
  Time Delay2/1 -> Stretch Reflex Left/3(v_ce)
  Time Delay1/1 -> Stretch Reflex Left/2(l_ce)
  Time Delay/1 -> Stretch Reflex Left/1(lambda)
  Time Delay4/1 -> Stretch Reflex Right/2(l_ce)
  Time Delay5/1 -> Stretch Reflex Right/3(v_ce)
  Time Delay3/1 -> Stretch Reflex Right/1(lambda)
  Saturation1/1 -> Activation Left/1
  Saturation4/1 -> Activation Right/1

== system ramadan_2022/Supraspinal Level/Finite State Machine ==
  note: Finite State Machine (FSM): The FSM comprises 4 states (Early Right Swing (0), Late Right Swing (1), Early Left Swing (2) and Late Left Swing (3)). The FSM transitions from state 0 to state 1 and from state 2 to state 3 when the time dt in state 0/2 is passed. It transitions from state 2 to state 3 and from state 3 to state 1 when right/left contact is measured.
  Information: Ground Contact : Inport
  Chart : Stateflow chart  TreatAsAtomicUnit=on
      settings: PortSchema="{\"entries\":[{\"content\":{\"sides\":[{\"content\":{\"connectorIds\":[\"In3\",\"In4\",\"In5\"]},\"type\":\"ConnectorPlacement.EquallySpacedRectSide\",\"uuid\":\"32e0668c-48c8-429f-a891-bfe2264b7e83\"},{\"content\":{\"connectorIds\":[\"Out1\",\"Out2\",\"Out3\",\"Out4\",\"Out5\",\"Out6\"],\"side\":\"RIGHT\"},\"type\":\"ConnectorPlacement.EquallySpacedRectSide\",\"uuid\":\"eb9fc1c2-0f15-47d7-b4d3-2749cce0de04\"},{\"content\":{\"connectorIds\":[\"In1\",\"In2\"],\"side\":\"TOP\"},\"type\":\"ConnectorPlacement.EquallySpacedRectSide\",\"uuid\":\"f1bd4247-3561-4736-9dd1-6be63b5db75c\"}]},\"type\":\"ConnectorPlacement.EquallySpacedConnector\",\"uuid\":\"7da9c37e-47e6-4ed1-b08d-da72e495dbd7\"}],\"packageUris\":[\"http://schema.mathworks.com/mf0/Connector/R2020b\"],\"version\":\"1.0\"}"
  Constant : Constant  Value=lp1
  Constant1 : Constant  Value=lp2
  Demux : Demux  Outputs=2
  Early Right Swing : Outport
  Late Right Swing : Outport  Port=2
  Early Left Swing : Outport  Port=3
  Late Left Swing : Outport  Port=4
  Landing Preparation Right : Outport  Port=5
  Landing Preparation Left : Outport  Port=6
  wires:
  Demux/1 -> Chart/4(contact_left)
  Demux/2 -> Chart/5(contact_right)
  Information: Ground Contact/1 -> Demux/1
  Chart/1(state0) -> Early Right Swing/1
  Chart/2(state1) -> Late Right Swing/1
  Chart/3(state2) -> Early Left Swing/1
  Chart/4(state3) -> Late Left Swing/1
  [step_dur] -> Chart/3(dt)
  Chart/5(state4) -> Landing Preparation Right/1
  Chart/6(state5) -> Landing Preparation Left/1
  Constant/1 -> Chart/2(lp1)
  Constant1/1 -> Chart/1(lp2)

== system ramadan_2022/Supraspinal Level/Subsystem ==
  note: Positive Forces
  note: Muscle Inversion
  note: Stretch Reflex Inversion
  Early/Late Swing : Inport
  Landing Preparation : Inport  Port=2
  Swing Right : Inport  Port=3
  Compute positives forces that generate desired torque profiles : Subsystem
  Inversion of Muscle Model : Subsystem
  NOT : Logic  Operator=NOT  AllPortsSameDT=off  OutDataTypeStr=boolean
  Product2 : Product
  Product3 : Product
  Scope : Scope
  Scope1 : Scope
  Stance Leg2 : Subsystem
  Stretch Reflex Inversion : Subsystem
  Swing Leg : Subsystem
  Terminator : Terminator
  Terminator1 : Terminator
  Descending Command Left : Outport
  Descending Command Right : Outport  Port=2
  wires:
  Swing Right/1 -> NOT/1, Product2/2, Compute positives forces that generate desired torque profiles/1(Left/Right), Stance Leg2/1(Left/Right), Swing Leg/1(Left/Right)
  Stretch Reflex Inversion/2(Descending Command Right) -> Descending Command Right/1
  Inversion of Muscle Model/1(Desired Activation Left) -> Stretch Reflex Inversion/1(Desired Activation Left)
  Stretch Reflex Inversion/1(Descending Command Left) -> Descending Command Left/1
  Inversion of Muscle Model/2(Desired Activation Right) -> Scope1/1, Stretch Reflex Inversion/2(Desired Activation Right)
  Early/Late Swing/1 -> Swing Leg/3(Early/Late Swing)
  Swing Leg/1(Desired Torques Left Swing) -> Compute positives forces that generate desired torque profiles/3(Swing Left)
  Swing Leg/2(Desired Torques Right Swing) -> Scope/1, Compute positives forces that generate desired torque profiles/4(Swing Right)
  Stance Leg2/1(Push Off Left) -> Product2/1
  Product2/1 -> Compute positives forces that generate desired torque profiles/2(Stance Left)
  Compute positives forces that generate desired torque profiles/1(Desired Force) -> Inversion of Muscle Model/1(Desired Forces)
  NOT/1 -> Product3/2
  Product3/1 -> Compute positives forces that generate desired torque profiles/5(Stance Right)
  Stance Leg2/2(Push Off Right) -> Product3/1
  Swing Leg/3(Interaction Torques Left) -> Terminator/1
  Swing Leg/4(Interaction Torques Right) -> Terminator1/1
  Landing Preparation/1 -> Swing Leg/2(Landing Preparation)

== system ramadan_2022/Body and Contact Model/L Leg/Ankle Mechanical Limits ==
  note: Overextension Torque
  note: Joint Limits
  note: Overflexion Torque
  dq [rad/s] : Inport
  q [rad] : Inport  Port=2
  Gain1 : Gain  Gain=mParams.joints.ankle.kStop
  Gain2 : Gain  Gain=-1
  Gain3 : Gain  Gain=mParams.joints.ankle.kStop
  Gain4 : Gain  Gain=1/mParams.joints.ankle.wMaxStop
  Gain5 : Gain  Gain=-1
  Gain6 : Gain  Gain=-1
  Limit Knee Range : simulink/Logic and Bit Operations/Interval Test  IntervalClosedRight=on  uplimit=mParams.joints.ankle.MaxPitch + 20*pi/180  IntervalClosedLeft=on  lowlimit=mParams.joints.ankle.MinPitch - 20*pi/180  OutDataTypeStr=boolean
      settings: AttributesFormatString=|
      | Lower limits: %<lowlimit>
      | Upper limits: %<uplimit>
  Logical Operator3 : Logic  Operator=NOT  AllPortsSameDT=off  OutDataTypeStr=boolean
  Product1 : Product  Inputs=4
  Product2 : Product  Inputs=4
  Stop Simulation1 : Stop
  Sum : Sum  Inputs=|+-
  Sum1 : Sum  Inputs=|+-
  Sum2 : Sum
  Sum3 : Sum  Inputs=|-+
  Sum4 : Sum  Inputs=|-+
  above upper limit? : simulink/Logic and Bit Operations/Compare To Zero  relop=>  OutDataTypeStr=boolean  ZeroCross=off
  below lower limit? : simulink/Logic and Bit Operations/Compare To Zero  relop=<  OutDataTypeStr=boolean  ZeroCross=off
  const : Constant
  const1 : Constant
  mech limit pushes back? : simulink/Logic and Bit Operations/Compare To Zero  relop=>  OutDataTypeStr=boolean  ZeroCross=off
  mech limit pushes back?. : simulink/Logic and Bit Operations/Compare To Zero  relop=>  OutDataTypeStr=boolean  ZeroCross=off
  overextension angle : Constant  Value=mParams.joints.ankle.MaxPitch
  overflexion angle : Constant  Value=mParams.joints.ankle.MinPitch
  tau [Nm] : Outport  VectorParamsAs1DForOutWhenUnconnected=off
  wires:
  Logical Operator3/1 -> Stop Simulation1/1
  Limit Knee Range/1 -> Logical Operator3/1
  Gain6/1 -> Sum2/1
  Gain2/1 -> Sum3/1
  Sum2/1 -> tau [Nm]/1
  overflexion angle/1 -> Sum1/2
  Sum1/1 -> Gain1/1
  Sum/1 -> Gain3/1
  q [rad]/1 -> Sum1/1, Limit Knee Range/1, Sum/1
  overextension angle/1 -> Sum/2
  dq [rad/s]/1 -> Gain4/1
  const/1 -> Sum3/2
  Sum3/1 -> Product1/3, mech limit pushes back?/1
  Gain3/1 -> Product1/2, above upper limit?/1
  mech limit pushes back?/1 -> Product1/4
  above upper limit?/1 -> Product1/1
  Product1/1 -> Gain6/1
  Product2/1 -> Gain5/1
  below lower limit?/1 -> Product2/1
  mech limit pushes back?./1 -> Product2/4
  Gain1/1 -> below lower limit?/1, Product2/2
  Sum4/1 -> mech limit pushes back?./1, Product2/3
  const1/1 -> Sum4/2
  Gain4/1 -> Sum4/1, Gain2/1
  Gain5/1 -> Sum2/2
